simulink model "DTP_PMSM_VSD_Four_Vector_Control"  (R2024b)
settings: Solver=ode3  StartTime=0.0  StopTime=0.2  FixedStep=1e-6  RelTol=1e-3
InitFcn:
  | Udc=100;
  | Kp_omega = 2;
  | Ki_omega = 0;
  | 
  | Kp_id = 0.008*550;
  | Ki_id = 1.4*550;
  | Kp_iq = 0.008*550;
  | Ki_iq = 1.4*550;
  | Kp_z  = 0.1;
  | Ki_z  = 0.0001;
  | 
  | Ts = 1e-4;
  | flux = 0.015;
  | Toff = 1.02;
model workspace (MAT data in the model file):
  B = 0
  J = 0.000118
  Ki_id = 770
  Ki_iq = 770
  Ki_omega = 0
  Ki_z = 0.0001
  Kp_id = 4.4
  Kp_iq = 4.4
  Kp_omega = 2
  Kp_z = 0.1
  Lm = 1e-05
  Ls = 0.0001
  Pn = 5
  Rs = 0.28
  Toff = 1.02
  Ts = 0.0001
  Vdc = 100
  flux = 0.015
libraries: spsControlledVoltageSourceLib x6, spsCurrentMeasurementLib x6, powerlib_extras x5, spsUniversalBridgeLib x2, spsMutualInductanceLib x1, spsGroundLib x1, spsDCVoltageSourceLib x1, spspowerguiLib x1, simulink x1
settings Model: Creator=zx  LastModifiedBy=31904
settings SolverCC: AlgebraicLoopSolver=TrustRegion
settings DataIOCC: ReturnWorkspaceOutputs=off
settings DebuggingCC: ArithmeticOperatorsInVariantConditions=warning
settings SFSimCC: CustomCodeUndefinedFunction=UseInterfaceOnly
settings RTWCC: GPUComputeCapability=3.5

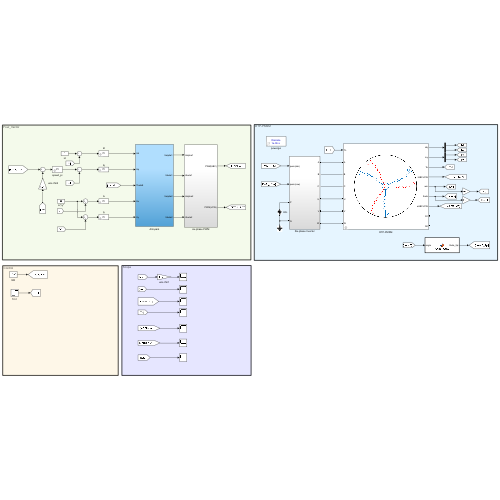
[thumbnail: Simulink's stored preview of the top-level diagram]
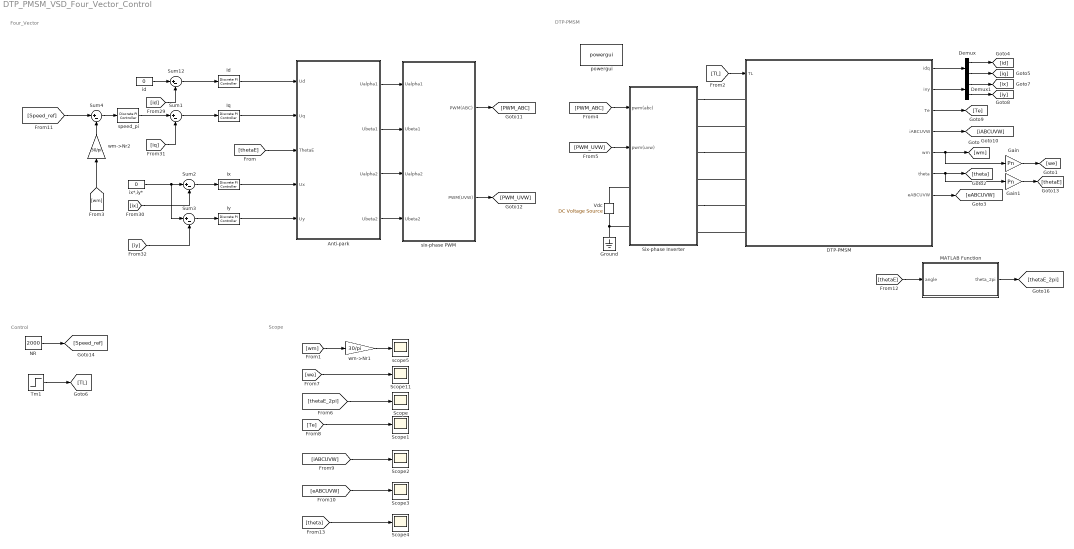
== system DTP_PMSM_VSD_Four_Vector_Control ==
  note: Four_Vector
  note: Control
  note: DTP-PMSM
  note: Scope
  Anti-park : Subsystem
  DTP-PMSM : Subsystem  mask{flux=flux, Ls=Ls, Lm=Lm, Rs=Rs, Inertia=J, Friction=B, Pairs=Pn}
      mask DialogControl ParameterGroupVar Prompt: DTP-PMSM Parameters
      mask Display: image('DTP-PMSM.png', [0,0,0,0,75,75]);
  Demux : Demux  Outputs=2
  Demux1 : Demux  Outputs=2
  Gain : Gain  Gain=Pn
  Gain1 : Gain  Gain=Pn
  Ground : spsGroundLib/Ground  LConnTagsString=a
  Id : powerlib_extras/Discrete  Control Blocks/Discrete PI Controller  Kp=0.111  Ki=280  Par_Limits=[Vdc*0.9*sqrt(1/3) -Vdc*0.9*sqrt(1/3)]  Init=0  Ts=Ts
  Iq : powerlib_extras/Discrete  Control Blocks/Discrete PI Controller  Kp=0.111  Ki=280  Par_Limits=[Vdc*0.9*sqrt(1/3) -Vdc*0.9*sqrt(1/3)]  Init=0  Ts=Ts
  Ix : powerlib_extras/Discrete  Control Blocks/Discrete PI Controller  Kp=Kp_z  Ki=Ki_z  Par_Limits=[100 -100]  Init=0  Ts=Ts
  Iy : powerlib_extras/Discrete  Control Blocks/Discrete PI Controller  Kp=Kp_z  Ki=Ki_z  Par_Limits=[100 -100]  Init=0  Ts=Ts
  MATLAB Function : MATLAB Function  TreatAsAtomicUnit=on
  NR : Constant  Value=2000
  Scope{,1..4,11} (6 alike) : Scope
  Six-phase Inverter : Subsystem
  Sum{1..4,12} (5 alike) : Sum  Inputs=|+-
  Tm1 : Step  Time=0.1  SampleTime=0
  Vdc : spsDCVoltageSourceLib/DC Voltage Source  Amplitude=Vdc  Measurements=None
  id : Constant  Value=0
  ix*,iy* : Constant  Value=0
  powergui : spspowerguiLib/powergui  Priority=1  SimulationMode=Discrete  SampleTime=1e-6  frequency=60  Iterations=50  frequencyindice=0  Pbase=100e6  ErrMax=1e-4  UnitsV=kV  UnitsW=MW  buscounter=0  FunctionMessages=off  echomessages=off  EnableUseOfTLC=off  CurrentSourceSwitches=off  DisableSnubberDevices=off  DisableRonSwitches=off  DisableVfSwitches=off  DisplayEquations=off  AutomaticDiscreteSolvers=off  SolverType=Tustin/Backward Euler (TBE)  Interpol=off  ExternalGateDelay=off  methode=off  Ts=100  x0status=blocks  SPID=on  SwTol=0  HookPort=off  NonlinearTolerance=1e-4  nMaxIteration=100  ContinueOnMaxIteration=off  RestoreLinks=warning  ResistiveCurrentMeasurement=off  Frange=[0:2:500]  Ylog=off  Xlog=on  ShowGrid=off  save=off  variable=ZData  structure=0  ZoomFFT=off  StartTime=0.0  cycles=1  DisplayStyle=1  fundamental=60  FreqAxis=off  MaxFrequency=1000  frequencyindicesteady=1  RmsSteady=1  display=off
  scope5 : Scope
  six-phase PWM : Subsystem
  speed_pi : powerlib_extras/Discrete  Control Blocks/Discrete PI Controller  Kp=0.03  Ki=1  Par_Limits=[50 -50]  Init=0  Ts=0.0001
  wm->Nr1 : Gain  Gain=30/pi
  wm->Nr2 : Gain  Gain=30/pi
  wires:
  [thetaE] -> Anti-park/3(ThetaE)
  Iq/1 -> Anti-park/2(Uq)
  [iq] -> Sum1/2
  id/1 -> Sum12/1
  Sum1/1 -> Iq/1
  Sum4/1 -> speed_pi/1
  Sum12/1 -> Id/1
  Ix/1 -> Anti-park/4(Ux)
  speed_pi/1 -> Sum1/1
  Id/1 -> Anti-park/1(Ud)
  Sum3/1 -> Iy/1
  NR/1 -> [Speed_ref]
  ix*,iy*/1 -> Sum3/1, Sum2/1
  Sum2/1 -> Ix/1
  Iy/1 -> Anti-park/5(Uy)
  [wm] -> wm->Nr2/1
  [wm] -> wm->Nr1/1
  wm->Nr1/1 -> scope5/1
  [ix] -> Sum2/2
  [iy] -> Sum3/2
  [id] -> Sum12/2
  Tm1/1 -> [TL]
  Anti-park/1(Ualpha1) -> six-phase PWM/1(Ualpha1)
  Anti-park/2(Ubeta1) -> six-phase PWM/2(Ubeta1)
  Anti-park/3(Ualpha2) -> six-phase PWM/3(Ualpha2)
  Anti-park/4(Ubeta2) -> six-phase PWM/4(Ubeta2)
  six-phase PWM/1(PWM(ABC)) -> [PWM_ABC]
  six-phase PWM/2(PWM(UVW)) -> [PWM_UVW]
  wm->Nr2/1 -> Sum4/2
  DTP-PMSM/4(iABCUVW) -> [iABCUVW]
  DTP-PMSM/3(Te) -> [Te]
  DTP-PMSM/2(ixy) -> Demux1/1
  DTP-PMSM/1(idq) -> Demux/1
  [we] -> Scope11/1
  DTP-PMSM/5(wm) -> Gain/1, [wm]
  Gain/1 -> [we]
  DTP-PMSM/6(theta) -> [theta], Gain1/1
  DTP-PMSM/7(eABCUVW) -> [eABCUVW]
  Demux/1 -> [id]
  Demux/2 -> [iq]
  [TL] -> DTP-PMSM/1(TL)
  Demux1/1 -> [ix]
  Demux1/2 -> [iy]
  [PWM_UVW] -> Six-phase Inverter/2(pwm(uvw))
  [PWM_ABC] -> Six-phase Inverter/1(pwm(abc))
  [Te] -> Scope1/1
  [iABCUVW] -> Scope2/1
  [eABCUVW] -> Scope3/1
  Gain1/1 -> [thetaE]
  [Speed_ref] -> Sum4/1
  [thetaE] -> MATLAB Function/1(angle)
  MATLAB Function/1(theta_2pi) -> [thetaE_2pi]
  [thetaE_2pi] -> Scope/1
  [theta] -> Scope4/1
  connections:
  DTP-PMSM/LConn4 -- Six-phase Inverter/RConn4
  Six-phase Inverter/RConn5 -- DTP-PMSM/LConn5
  Six-phase Inverter/RConn3 -- DTP-PMSM/LConn3
  DTP-PMSM/LConn2 -- Six-phase Inverter/RConn2
  Six-phase Inverter/RConn1 -- DTP-PMSM/LConn1
  DTP-PMSM/LConn6 -- Six-phase Inverter/RConn6
  Vdc/RConn1 -- Six-phase Inverter/LConn1
  Six-phase Inverter/LConn2 -- Vdc/LConn1 -- Ground/LConn1

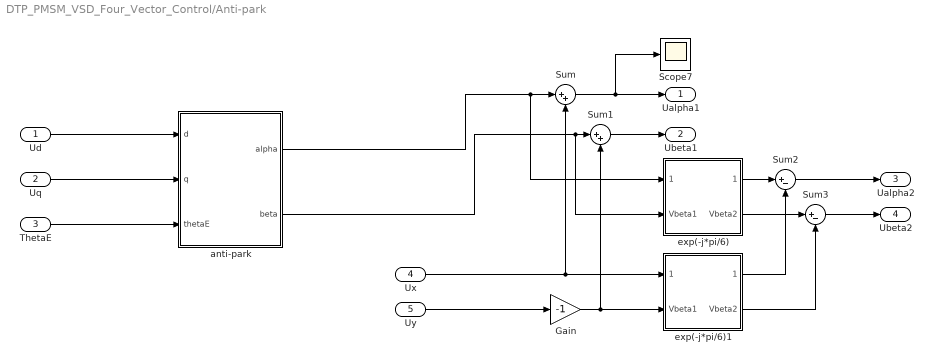
== system DTP_PMSM_VSD_Four_Vector_Control/Anti-park ==
  Ud : Inport
  Uq : Inport  Port=2
  ThetaE : Inport  Port=3
  Ux : Inport  Port=4
  Uy : Inport  Port=5
  Gain : Gain  Gain=-1
  Scope7 : Scope
  Sum : Sum  Inputs=|++
  Sum1 : Sum  Inputs=|++
  Sum2 : Sum  Inputs=|+-
  Sum3 : Sum  Inputs=|+-
  anti-park : Subsystem
      mask Display: disp('anti-park')
  exp(-j*pi/6) : Subsystem
  exp(-j*pi/6)1 : Subsystem
  Ualpha1 : Outport  VectorParamsAs1DForOutWhenUnconnected=off
  Ubeta1 : Outport  Port=2  VectorParamsAs1DForOutWhenUnconnected=off
  Ualpha2 : Outport  Port=3  VectorParamsAs1DForOutWhenUnconnected=off
  Ubeta2 : Outport  Port=4  VectorParamsAs1DForOutWhenUnconnected=off
  wires:
  ThetaE/1 -> anti-park/3(thetaE)
  Ud/1 -> anti-park/1(d)
  Uq/1 -> anti-park/2(q)
  Sum1/1 -> Ubeta1/1
  Sum3/1 -> Ubeta2/1
  Sum/1 -> Scope7/1, Ualpha1/1
  Sum2/1 -> Ualpha2/1
  Ux/1 -> Sum/2, exp(-j*pi/6)1/1(Valpha1)
  anti-park/2(beta) -> exp(-j*pi/6)/2(Vbeta1), Sum1/1
  exp(-j*pi/6)/2(Vbeta2) -> Sum3/1
  Gain/1 -> Sum1/2, exp(-j*pi/6)1/2(Vbeta1)
  Uy/1 -> Gain/1
  exp(-j*pi/6)/1(Valpha2) -> Sum2/1
  exp(-j*pi/6)1/1(Valpha2) -> Sum2/2
  exp(-j*pi/6)1/2(Vbeta2) -> Sum3/2
  anti-park/1(alpha) -> exp(-j*pi/6)/1(Valpha1), Sum/1

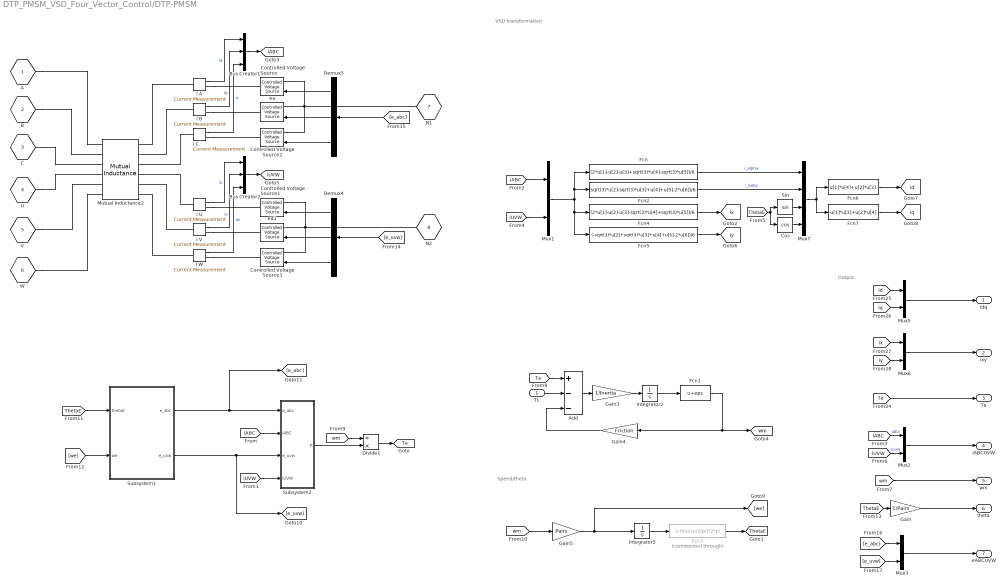
== system DTP_PMSM_VSD_Four_Vector_Control/DTP-PMSM ==
  note: Speed/theta
  note: Output
  note: VSD transformation
  TL : Inport
  Add : Sum  Inputs=+--
  Bus Creator1 : BusCreator  Inputs=3
  Bus Creator2 : BusCreator  Inputs=3
  Controlled Voltage Source{,1..3} (4 alike) : spsControlledVoltageSourceLib/Controlled Voltage Source  Initialize=on  Source_Type=AC  Amplitude=0  Phase=0  Frequency=0  Measurements=None
  Cos : Trigonometry  Operator=cos
  Demux3 : Demux  Outputs=3
  Demux4 : Demux  Outputs=3
  Divide1 : Product  Inputs=/*
  Fcn : Fcn  Expr=(2*u[1]-u[2]-u[3]+sqrt(3)*u[4]-sqrt(3)*u[5])/6
  Fcn1 : Fcn  Expr=u+eps
  Fcn2 : Fcn  Expr=(sqrt(3)*u[2]-sqrt(3)*u[3]+u[4]+u[5]-2*u[6])/6
  Fcn3 : Fcn  Commented=through  Expr=u-floor(u/2/pi)*2*pi
  Fcn4 : Fcn  Expr=(2*u[1]-u[2]-u[3]-sqrt(3)*u[4]+sqrt(3)*u[5])/6
  Fcn5 : Fcn  Expr=(-sqrt(3)*u[2]+sqrt(3)*u[3]+u[4]+u[5]-2*u[6])/6
  Fcn6 : Fcn  Expr=u[1]*u[4]+u[2]*u[3]
  Fcn7 : Fcn  Expr=-u[1]*u[3]+u[2]*u[4]
  Gain : Gain  Gain=1/Pairs
  Gain3 : Gain  Gain=1/Inertia
  Gain4 : Gain  Gain=Friction
  Gain5 : Gain  Gain=Pairs
  I A : spsCurrentMeasurementLib/Current Measurement  PhasorSimulation=off  OutputType=Complex  PSBequivalent=0
  I B : spsCurrentMeasurementLib/Current Measurement  PhasorSimulation=off  OutputType=Complex  PSBequivalent=0
  I C : spsCurrentMeasurementLib/Current Measurement  PhasorSimulation=off  OutputType=Complex  PSBequivalent=0
  I U : spsCurrentMeasurementLib/Current Measurement  PhasorSimulation=off  OutputType=Complex  PSBequivalent=0
  I V : spsCurrentMeasurementLib/Current Measurement  PhasorSimulation=off  OutputType=Complex  PSBequivalent=0
  I W : spsCurrentMeasurementLib/Current Measurement  PhasorSimulation=off  OutputType=Complex  PSBequivalent=0
  Integrator2 : Integrator  UpperSaturationLimit=100  LowerSaturationLimit=-100
  Integrator3 : Integrator
  Mutual Inductance2 : spsMutualInductanceLib/Mutual Inductance  LConnTagsString=a|b|c|L4|L5|L6  RConnTagsString=A|B|C|R4|R5|R6  TypeOfMutual=Generalized mutual inductance  NumberOfWindings=6  SelfImpedance1=[0.306 0.0016]  SelfImpedance2=[0.306 0.0016]  ThreeWindings=on  SelfImpedance3=[0.306 0.0016]  MutualImpedance=[0 0.0008]  InductanceMatrix=[Ls -Lm -Lm 1.732508*Lm -1.732508*Lm 0; -Lm Ls -Lm 0 1.732508*Lm -1.732508*Lm; -Lm -Lm Ls -1.732508*Lm 0 1.732508*Lm; 1.732508*Lm 0 -1.732508*Lm Ls -Lm -Lm; -1.732508*Lm 1.732508*Lm 0 -Lm Ls -Lm; 0 -1.732508*Lm 1.732508*Lm -Lm -Lm Ls]  ResistanceMatrix=[Rs 0 0 0 0 0; 0 Rs 0 0 0 0; 0 0 Rs 0 0 0; 0 0 0 Rs 0 0; 0 0 0 0 Rs 0; 0 0 0 0 0 Rs]  Measurements=None
      settings: LibrarySourceBlock=sps_lib/Passives/Mutual Inductance
  Mux{1..3,5..6} (5 alike) : Mux  Inputs=2
  Mux7 : Mux
  Sin : Trigonometry
  Subsystem1 : Subsystem
  Subsystem2 : Subsystem
  ea : spsControlledVoltageSourceLib/Controlled Voltage Source  Initialize=on  Source_Type=AC  Amplitude=0  Phase=0  Frequency=0  Measurements=None
  ea1 : spsControlledVoltageSourceLib/Controlled Voltage Source  Initialize=on  Source_Type=AC  Amplitude=0  Phase=0  Frequency=0  Measurements=None
  A : PMIOPort  Side=Left
  B : PMIOPort  Port=2  Side=Left
  C : PMIOPort  Port=3  Side=Left
  U : PMIOPort  Port=4  Side=Left
  V : PMIOPort  Port=5  Side=Left
  W : PMIOPort  Port=6  Side=Left
  N1 : PMIOPort  Port=7  Side=Right
  N2 : PMIOPort  Port=8  Side=Right
  idq : Outport  VectorParamsAs1DForOutWhenUnconnected=off
  ixy : Outport  Port=2  VectorParamsAs1DForOutWhenUnconnected=off
  Te : Outport  Port=3  VectorParamsAs1DForOutWhenUnconnected=off
  iABCUVW : Outport  Port=4  VectorParamsAs1DForOutWhenUnconnected=off
  wm : Outport  Port=5  VectorParamsAs1DForOutWhenUnconnected=off
  theta : Outport  Port=6  VectorParamsAs1DForOutWhenUnconnected=off
  eABCUVW : Outport  Port=7  VectorParamsAs1DForOutWhenUnconnected=off
  tag scope: Te=global, ThetaE=global, iABC=global, iUVW=global, id=global, iq=global, ix=global, iy=global, wm=global
  wires:
  Subsystem1/1(e_abc) -> [e_abc], Subsystem2/1(e_abc)
  Subsystem1/2(e_uvw) -> [e_uvw], Subsystem2/3(e_uvw)
  Demux3/1 -> Controlled Voltage Source/1
  Demux3/2 -> ea/1
  Demux3/3 -> Controlled Voltage Source2/1
  Demux4/1 -> Controlled Voltage Source1/1
  Demux4/2 -> ea1/1
  Demux4/3 -> Controlled Voltage Source3/1
  I A/1 -> Bus Creator1/1  "ia"
  I B/1 -> Bus Creator1/2  "ib"
  I C/1 -> Bus Creator1/3  "ic"
  I U/1 -> Bus Creator2/1  "iu"
  I V/1 -> Bus Creator2/2  "iv"
  I W/1 -> Bus Creator2/3  "iw"
  Bus Creator1/1 -> [iABC]
  Bus Creator2/1 -> [iUVW]
  [iABC] -> Subsystem2/2(iABC)
  [iUVW] -> Subsystem2/4(iUVW)
  Subsystem2/1(P) -> Divide1/2
  Divide1/1 -> [Te]
  TL/1 -> Add/2
  Add/1 -> Gain3/1
  Gain3/1 -> Integrator2/1
  Integrator2/1 -> Fcn1/1
  Fcn1/1 -> [wm], Gain4/1
  Gain4/1 -> Add/3
  Gain5/1 -> [we], Integrator3/1
  Integrator3/1 -> Fcn3/1
  Fcn3/1 -> [ThetaE]
  Fcn4/1 -> [ix]
  Mux1/1 -> Fcn2/1, Fcn/1, Fcn4/1, Fcn5/1
  [iUVW] -> Mux1/2
  Fcn7/1 -> [iq]
  [iABC] -> Mux1/1
  [ThetaE] -> Sin/1, Cos/1
  Fcn5/1 -> [iy]
  Fcn6/1 -> [id]
  Mux7/1 -> Fcn6/1, Fcn7/1
  Fcn2/1 -> Mux7/2  "i_beta"
  Fcn/1 -> Mux7/1  "i_alpha"
  Cos/1 -> Mux7/4
  Sin/1 -> Mux7/3
  Mux5/1 -> idq/1
  [id] -> Mux5/1
  Mux6/1 -> ixy/1
  [iy] -> Mux6/2
  [ix] -> Mux6/1
  [iq] -> Mux5/2
  [Te] -> Te/1
  [iABC] -> Mux2/1  "iabc"
  [iUVW] -> Mux2/2  "iuvw"
  [wm] -> wm/1
  Mux2/1 -> iABCUVW/1
  [Te] -> Add/1
  [wm] -> Divide1/1
  [wm] -> Gain5/1
  [ThetaE] -> Subsystem1/1(thetaE)
  [we] -> Subsystem1/2(we)
  [ThetaE] -> Gain/1
  Gain/1 -> theta/1
  [e_uvw] -> Demux4/1
  [e_abc] -> Demux3/1
  [e_abc] -> Mux3/1
  [e_uvw] -> Mux3/2
  Mux3/1 -> eABCUVW/1
  connections:
  N1/RConn1 -- Controlled Voltage Source/LConn1 -- ea/LConn1 -- Controlled Voltage Source2/LConn1
  I C/LConn1 -- Mutual Inductance2/RConn3
  A/RConn1 -- Mutual Inductance2/LConn1
  B/RConn1 -- Mutual Inductance2/LConn2
  C/RConn1 -- Mutual Inductance2/LConn3
  I B/RConn1 -- ea/RConn1
  I A/RConn1 -- Controlled Voltage Source/RConn1
  I B/LConn1 -- Mutual Inductance2/RConn2
  I C/RConn1 -- Controlled Voltage Source2/RConn1
  I A/LConn1 -- Mutual Inductance2/RConn1
  I U/RConn1 -- Controlled Voltage Source1/RConn1
  U/RConn1 -- Mutual Inductance2/LConn4
  I W/RConn1 -- Controlled Voltage Source3/RConn1
  I U/LConn1 -- Mutual Inductance2/RConn4
  I V/LConn1 -- Mutual Inductance2/RConn5
  Controlled Voltage Source3/LConn1 -- Controlled Voltage Source1/LConn1 -- ea1/LConn1 -- N2/RConn1
  V/RConn1 -- Mutual Inductance2/LConn5
  I V/RConn1 -- ea1/RConn1
  I W/LConn1 -- Mutual Inductance2/RConn6
  W/RConn1 -- Mutual Inductance2/LConn6

== system DTP_PMSM_VSD_Four_Vector_Control/Six-phase Inverter ==
  pwm(abc) : Inport
  pwm(uvw) : Inport  Port=2
  Universal Bridge : spsUniversalBridgeLib/Universal Bridge  Arms=3  SnubberResistance=1e5  SnubberCapacitance=inf  Device=IGBT / Diodes  Ron=1e-3  Lon=0  ForwardVoltages="[  0  0  ]"  ForwardVoltage=0  GTOparameters=[ 10e-6 , 20e-6 ]  IGBTparameters=[ 1e-6 , 2e-6 ]  Measurements=None  Measurements_2=None  converterType=Rectifier
  Universal Bridge1 : spsUniversalBridgeLib/Universal Bridge  Arms=3  SnubberResistance=1e5  SnubberCapacitance=inf  Device=IGBT / Diodes  Ron=1e-3  Lon=0  ForwardVoltages="[  0  0  ]"  ForwardVoltage=0  GTOparameters=[ 10e-6 , 20e-6 ]  IGBTparameters=[ 1e-6 , 2e-6 ]  Measurements=None  Measurements_2=None  converterType=Rectifier
  A : PMIOPort  Side=Right
  B : PMIOPort  Port=2  Side=Right
  C : PMIOPort  Port=3  Side=Right
  U : PMIOPort  Port=4  Side=Right
  V : PMIOPort  Port=5  Side=Right
  W : PMIOPort  Port=6  Side=Right
  P : PMIOPort  Port=7  Side=Left
  N : PMIOPort  Port=8  Side=Left
  wires:
  pwm(uvw)/1 -> Universal Bridge/1
  pwm(abc)/1 -> Universal Bridge1/1
  connections:
  Universal Bridge/RConn2 -- N/RConn1 -- Universal Bridge1/RConn2
  Universal Bridge/RConn1 -- P/RConn1 -- Universal Bridge1/RConn1
  V/RConn1 -- Universal Bridge/LConn2
  U/RConn1 -- Universal Bridge/LConn1
  B/RConn1 -- Universal Bridge1/LConn2
  W/RConn1 -- Universal Bridge/LConn3
  C/RConn1 -- Universal Bridge1/LConn3
  A/RConn1 -- Universal Bridge1/LConn1

== system DTP_PMSM_VSD_Four_Vector_Control/six-phase PWM ==
  Ualpha1 : Inport
  Ubeta1 : Inport  Port=2
  Ualpha2 : Inport  Port=3
  Ubeta2 : Inport  Port=4
  Repeating Sequence : simulink/Sources/Repeating Sequence  rep_seq_t=[0 Ts/2 Ts]  rep_seq_y=[0 Ts/2 0]
  SVPWM : Subsystem
  SVPWM1 : Subsystem
  PWM(ABC) : Outport
  PWM(UVW) : Outport  Port=2
  wires:
  SVPWM/1(Pulse) -> PWM(ABC)/1
  Ubeta1/1 -> SVPWM/2(Ubeta)
  Ualpha2/1 -> SVPWM1/1(Ualpha)
  SVPWM1/1(Pulse) -> PWM(UVW)/1
  Repeating Sequence/1 -> SVPWM/3(Carrier wave), SVPWM1/3(Carrier wave)
  Ualpha1/1 -> SVPWM/1(Ualpha)
  Ubeta2/1 -> SVPWM1/2(Ubeta)

== system DTP_PMSM_VSD_Four_Vector_Control/Anti-park/anti-park ==
  d : Inport
  q : Inport  Port=2
  thetaE : Inport  Port=3
  Fcn : Fcn  Expr=u[1]*u[4]-u[2]*u[3]
  Fcn1 : Fcn  Expr=u[1]*u[3]+u[2]*u[4]
  Mux2 : Mux
  cos : Trigonometry  Operator=cos
  sin : Trigonometry
  alpha : Outport  VectorParamsAs1DForOutWhenUnconnected=off
  beta : Outport  Port=2  VectorParamsAs1DForOutWhenUnconnected=off
  wires:
  d/1 -> Mux2/1
  sin/1 -> Mux2/3
  Mux2/1 -> Fcn1/1, Fcn/1
  q/1 -> Mux2/2
  thetaE/1 -> sin/1, cos/1
  Fcn1/1 -> beta/1
  cos/1 -> Mux2/4
  Fcn/1 -> alpha/1

== system DTP_PMSM_VSD_Four_Vector_Control/Anti-park/exp(-j*pi//6) ==
  Valpha1 : Inport
  Vbeta1 : Inport  Port=2
  Fcn : Fcn  Expr=u(1)*cos(pi/6)+u(2)*sin(pi/6)
  Fcn1 : Fcn  Expr=-u(1)*sin(pi/6)+u(2)*cos(pi/6)
  Mux : Mux  Inputs=2
  Valpha2 : Outport  VectorParamsAs1DForOutWhenUnconnected=off
  Vbeta2 : Outport  Port=2  VectorParamsAs1DForOutWhenUnconnected=off
  wires:
  Vbeta1/1 -> Mux/2
  Valpha1/1 -> Mux/1
  Mux/1 -> Fcn1/1, Fcn/1
  Fcn/1 -> Valpha2/1
  Fcn1/1 -> Vbeta2/1

== system DTP_PMSM_VSD_Four_Vector_Control/Anti-park/exp(-j*pi//6)1 ==
  Valpha1 : Inport
  Vbeta1 : Inport  Port=2
  Fcn : Fcn  Expr=u(1)*cos(pi/6)+u(2)*sin(pi/6)
  Fcn1 : Fcn  Expr=-u(1)*sin(pi/6)+u(2)*cos(pi/6)
  Mux : Mux  Inputs=2
  Valpha2 : Outport  VectorParamsAs1DForOutWhenUnconnected=off
  Vbeta2 : Outport  Port=2  VectorParamsAs1DForOutWhenUnconnected=off
  wires:
  Vbeta1/1 -> Mux/2
  Valpha1/1 -> Mux/1
  Mux/1 -> Fcn1/1, Fcn/1
  Fcn/1 -> Valpha2/1
  Fcn1/1 -> Vbeta2/1

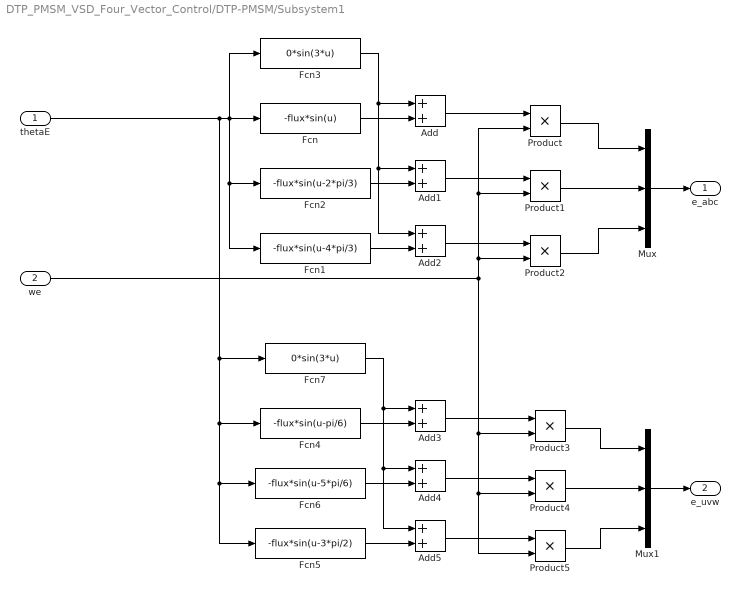
== system DTP_PMSM_VSD_Four_Vector_Control/DTP-PMSM/Subsystem1 ==
  thetaE : Inport
  we : Inport  Port=2
  Add{,1..5} (6 alike) : Sum
  Fcn : Fcn  Expr=-flux*sin(u)
  Fcn1 : Fcn  Expr=-flux*sin(u-4*pi/3)
  Fcn2 : Fcn  Expr=-flux*sin(u-2*pi/3)
  Fcn3 : Fcn  Expr=0*sin(3*u)
  Fcn4 : Fcn  Expr=-flux*sin(u-pi/6)
  Fcn5 : Fcn  Expr=-flux*sin(u-3*pi/2)
  Fcn6 : Fcn  Expr=-flux*sin(u-5*pi/6)
  Fcn7 : Fcn  Expr=0*sin(3*u)
  Mux : Mux  Inputs=3
  Mux1 : Mux  Inputs=3
  Product{,1..5} (6 alike) : Product
  e_abc : Outport
  e_uvw : Outport  Port=2
  wires:
  Product1/1 -> Mux/2
  Product2/1 -> Mux/3
  Mux/1 -> e_abc/1
  Product/1 -> Mux/1
  Fcn/1 -> Add/2
  Add/1 -> Product/1
  Fcn2/1 -> Add1/2
  Add1/1 -> Product1/1
  Fcn1/1 -> Add2/2
  Add2/1 -> Product2/1
  Fcn3/1 -> Add2/1, Add1/1, Add/1
  Product3/1 -> Mux1/1
  we/1 -> Product3/2, Product4/2, Product5/2, Product1/2, Product/2, Product2/2
  Product5/1 -> Mux1/3
  Add5/1 -> Product5/1
  Add4/1 -> Product4/1
  thetaE/1 -> Fcn5/1, Fcn6/1, Fcn4/1, Fcn7/1, Fcn1/1, Fcn2/1, Fcn3/1, Fcn/1
  Add3/1 -> Product3/1
  Fcn6/1 -> Add4/2
  Fcn4/1 -> Add3/2
  Product4/1 -> Mux1/2
  Fcn7/1 -> Add5/1, Add4/1, Add3/1
  Mux1/1 -> e_uvw/1
  Fcn5/1 -> Add5/2

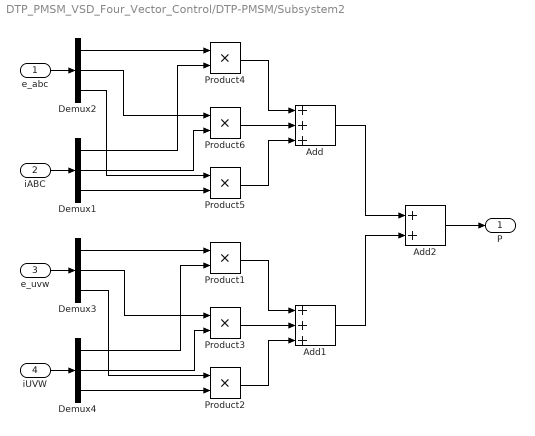
== system DTP_PMSM_VSD_Four_Vector_Control/DTP-PMSM/Subsystem2 ==
  e_abc : Inport
  iABC : Inport  Port=2
  e_uvw : Inport  Port=3
  iUVW : Inport  Port=4
  Add : Sum  Inputs=+++
  Add1 : Sum  Inputs=+++
  Add2 : Sum
  Demux{1..4} (4 alike) : Demux  Outputs=3
  Product{1..6} (6 alike) : Product
  P : Outport
  wires:
  e_abc/1 -> Demux2/1
  iABC/1 -> Demux1/1
  e_uvw/1 -> Demux3/1
  iUVW/1 -> Demux4/1
  Demux2/1 -> Product4/1
  Demux1/1 -> Product4/2
  Demux2/2 -> Product6/1
  Demux1/2 -> Product6/2
  Demux2/3 -> Product5/1
  Demux1/3 -> Product5/2
  Demux3/1 -> Product1/1
  Demux3/2 -> Product3/1
  Demux3/3 -> Product2/1
  Demux4/1 -> Product1/2
  Demux4/2 -> Product3/2
  Demux4/3 -> Product2/2
  Product6/1 -> Add/2
  Product4/1 -> Add/1
  Product5/1 -> Add/3
  Product3/1 -> Add1/2
  Product1/1 -> Add1/1
  Product2/1 -> Add1/3
  Add/1 -> Add2/1
  Add1/1 -> Add2/2
  Add2/1 -> P/1

== system DTP_PMSM_VSD_Four_Vector_Control/six-phase PWM/SVPWM ==
  Ualpha : Inport
  Ubeta : Inport  Port=2
  Carrier wave : Inport  Port=3
  PWM : Subsystem
  Sector Caculate : Subsystem
  T1T2 Caculate : Subsystem
  Tcm Caculate : Subsystem
  Tpwm : Constant  Value=Ts
  Vdc : Constant  Value=Vdc
  XYZ Caculate : Subsystem
  Pulse : Outport  VectorParamsAs1DForOutWhenUnconnected=off
  wires:
  Tcm Caculate/1(Tcm123) -> PWM/2(Tcm123)
  Carrier wave/1 -> PWM/1(In)
  PWM/1(PWM) -> Pulse/1
  Vdc/1 -> XYZ Caculate/4(Udc)
  Tpwm/1 -> XYZ Caculate/3(Ts), T1T2 Caculate/3(Tpwm), Tcm Caculate/4(Tpwm)
  T1T2 Caculate/2(T2) -> Tcm Caculate/3(T2)
  T1T2 Caculate/1(T1) -> Tcm Caculate/2(T1)
  XYZ Caculate/1(XYZ) -> T1T2 Caculate/2(XYZ)
  Sector Caculate/1(N) -> T1T2 Caculate/1(N), Tcm Caculate/1(N)
  Ubeta/1 -> Sector Caculate/2(Ubeta), XYZ Caculate/2(Ubeta)
  Ualpha/1 -> Sector Caculate/1(Ualpha), XYZ Caculate/1(Ualpha)

== system DTP_PMSM_VSD_Four_Vector_Control/six-phase PWM/SVPWM1 ==
  Ualpha : Inport
  Ubeta : Inport  Port=2
  Carrier wave : Inport  Port=3
  PWM : Subsystem
  Sector Caculate : Subsystem
  T1T2 Caculate : Subsystem
  Tcm Caculate : Subsystem
  Tpwm : Constant  Value=Ts
  Vdc : Constant  Value=Vdc
  XYZ Caculate : Subsystem
  Pulse : Outport  VectorParamsAs1DForOutWhenUnconnected=off
  wires:
  Tcm Caculate/1(Tcm123) -> PWM/2(Tcm123)
  Carrier wave/1 -> PWM/1(In)
  Ualpha/1 -> XYZ Caculate/1(Ualpha), Sector Caculate/1(Ualpha)
  Ubeta/1 -> XYZ Caculate/2(Ubeta), Sector Caculate/2(Ubeta)
  Sector Caculate/1(N) -> Tcm Caculate/1(N), T1T2 Caculate/1(N)
  XYZ Caculate/1(XYZ) -> T1T2 Caculate/2(XYZ)
  T1T2 Caculate/1(T1) -> Tcm Caculate/2(T1)
  T1T2 Caculate/2(T2) -> Tcm Caculate/3(T2)
  Tpwm/1 -> Tcm Caculate/4(Tpwm), T1T2 Caculate/3(Tpwm), XYZ Caculate/3(Ts)
  Vdc/1 -> XYZ Caculate/4(Udc)
  PWM/1(PWM) -> Pulse/1

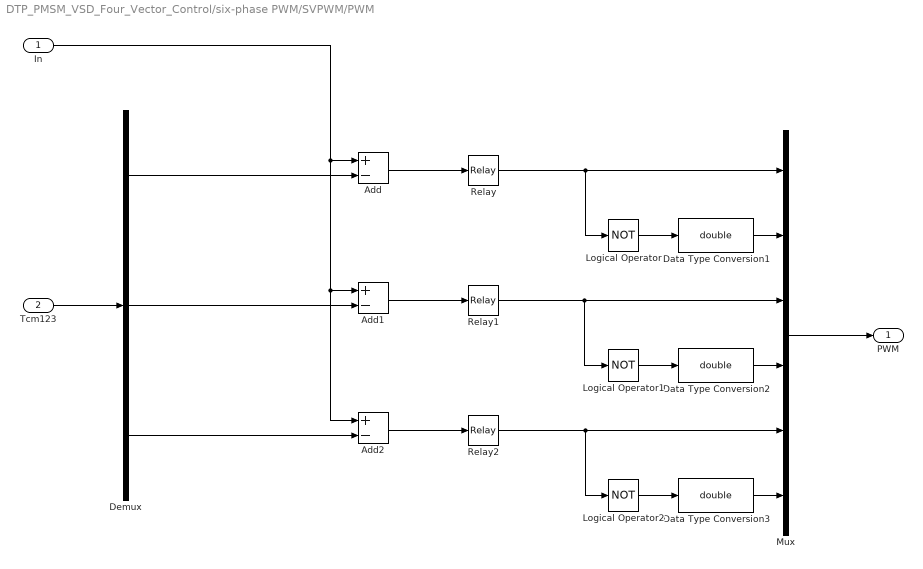
== system DTP_PMSM_VSD_Four_Vector_Control/six-phase PWM/SVPWM/PWM ==
  In : Inport
  Tcm123 : Inport  Port=2
  Add : Sum  Inputs=+-
  Add1 : Sum  Inputs=+-
  Add2 : Sum  Inputs=+-
  Data Type Conversion1 : DataTypeConversion  OutDataTypeStr=double
  Data Type Conversion2 : DataTypeConversion  OutDataTypeStr=double
  Data Type Conversion3 : DataTypeConversion  OutDataTypeStr=double
  Demux : Demux  Outputs=3
  Logical Operator : Logic  Operator=NOT  AllPortsSameDT=off  OutDataTypeStr=boolean
  Logical Operator1 : Logic  Operator=NOT  AllPortsSameDT=off  OutDataTypeStr=boolean
  Logical Operator2 : Logic  Operator=NOT  AllPortsSameDT=off  OutDataTypeStr=boolean
  Mux : Mux  Inputs=6
  Relay : Relay
  Relay1 : Relay
  Relay2 : Relay
  PWM : Outport  VectorParamsAs1DForOutWhenUnconnected=off
  wires:
  Data Type Conversion3/1 -> Mux/6
  Logical Operator2/1 -> Data Type Conversion3/1
  Data Type Conversion2/1 -> Mux/4
  Logical Operator1/1 -> Data Type Conversion2/1
  Data Type Conversion1/1 -> Mux/2
  Logical Operator/1 -> Data Type Conversion1/1
  Demux/3 -> Add2/2
  Demux/2 -> Add1/2
  Demux/1 -> Add/2
  Relay2/1 -> Logical Operator2/1, Mux/5
  Relay1/1 -> Mux/3, Logical Operator1/1
  Relay/1 -> Logical Operator/1, Mux/1
  Tcm123/1 -> Demux/1
  Add2/1 -> Relay2/1
  Add1/1 -> Relay1/1
  Add/1 -> Relay/1
  Mux/1 -> PWM/1
  In/1 -> Add1/1, Add2/1, Add/1

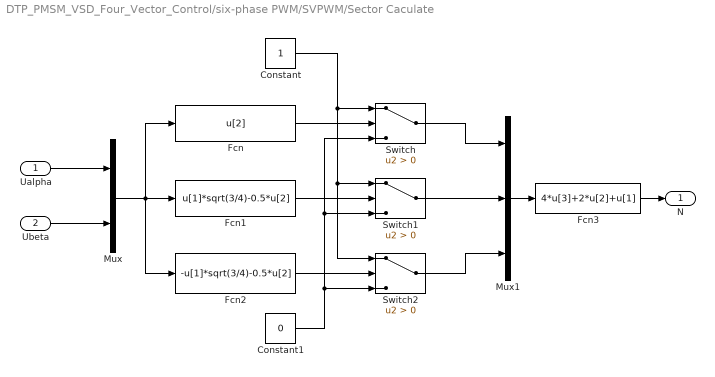
== system DTP_PMSM_VSD_Four_Vector_Control/six-phase PWM/SVPWM/Sector Caculate ==
  Ualpha : Inport
  Ubeta : Inport  Port=2
  Constant : Constant
  Constant1 : Constant  Value=0
  Fcn : Fcn  Expr=u[2]
  Fcn1 : Fcn  Expr=u[1]*sqrt(3/4)-0.5*u[2]
  Fcn2 : Fcn  Expr=-u[1]*sqrt(3/4)-0.5*u[2]
  Fcn3 : Fcn  Expr=4*u[3]+2*u[2]+u[1]
  Mux : Mux  Inputs=2
  Mux1 : Mux  Inputs=3
  Switch : Switch  Criteria=u2 > Threshold  SaturateOnIntegerOverflow=off  InputSameDT=off
  Switch1 : Switch  Criteria=u2 > Threshold  SaturateOnIntegerOverflow=off  InputSameDT=off
  Switch2 : Switch  Criteria=u2 > Threshold  SaturateOnIntegerOverflow=off  InputSameDT=off
  N : Outport  VectorParamsAs1DForOutWhenUnconnected=off
  wires:
  Constant1/1 -> Switch2/3, Switch1/3, Switch/3
  Constant/1 -> Switch/1, Switch2/1, Switch1/1
  Fcn2/1 -> Switch2/2
  Fcn1/1 -> Switch1/2
  Fcn/1 -> Switch/2
  Mux/1 -> Fcn/1, Fcn1/1, Fcn2/1
  Switch/1 -> Mux1/1
  Switch2/1 -> Mux1/3
  Switch1/1 -> Mux1/2
  Mux1/1 -> Fcn3/1
  Fcn3/1 -> N/1
  Ubeta/1 -> Mux/2
  Ualpha/1 -> Mux/1

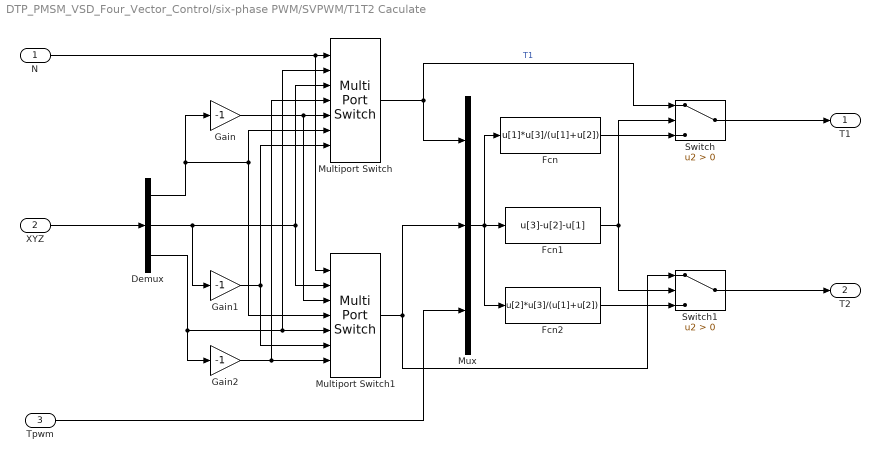
== system DTP_PMSM_VSD_Four_Vector_Control/six-phase PWM/SVPWM/T1T2 Caculate ==
  N : Inport
  XYZ : Inport  Port=2
  Tpwm : Inport  Port=3
  Demux : Demux  Outputs=3
  Fcn : Fcn  Expr=u[1]*u[3]/(u[1]+u[2])
  Fcn1 : Fcn  Expr=u[3]-u[2]-u[1]
  Fcn2 : Fcn  Expr=u[2]*u[3]/(u[1]+u[2])
  Gain : Gain  Gain=-1
  Gain1 : Gain  Gain=-1
  Gain2 : Gain  Gain=-1
  Multiport Switch : MultiPortSwitch  Inputs=6  DiagnosticForDefault=None  SaturateOnIntegerOverflow=off  InputSameDT=off
  Multiport Switch1 : MultiPortSwitch  Inputs=6  DiagnosticForDefault=None  SaturateOnIntegerOverflow=off  InputSameDT=off
  Mux : Mux  Inputs=3
  Switch : Switch  Criteria=u2 > Threshold  SaturateOnIntegerOverflow=off  InputSameDT=off
  Switch1 : Switch  Criteria=u2 > Threshold  SaturateOnIntegerOverflow=off  InputSameDT=off
  T1 : Outport  VectorParamsAs1DForOutWhenUnconnected=off
  T2 : Outport  Port=2  VectorParamsAs1DForOutWhenUnconnected=off
  wires:
  Switch1/1 -> T2/1
  Fcn2/1 -> Switch1/3
  Fcn1/1 -> Switch/2, Switch1/2
  Mux/1 -> Fcn/1, Fcn1/1, Fcn2/1
  Switch/1 -> T1/1
  Fcn/1 -> Switch/3
  Gain/1 -> Multiport Switch1/3, Multiport Switch/5
  Gain1/1 -> Multiport Switch/7, Multiport Switch1/6
  Gain2/1 -> Multiport Switch1/7, Multiport Switch/4
  Multiport Switch/1 -> Switch/1, Mux/1  "T1"
  Multiport Switch1/1 -> Mux/2, Switch1/1
  Tpwm/1 -> Mux/3
  Demux/3 -> Multiport Switch1/5, Multiport Switch/2, Gain2/1
  Demux/1 -> Multiport Switch/6, Multiport Switch1/4, Gain/1
  N/1 -> Multiport Switch/1, Multiport Switch1/1
  Demux/2 -> Gain1/1, Multiport Switch/3, Multiport Switch1/2
  XYZ/1 -> Demux/1

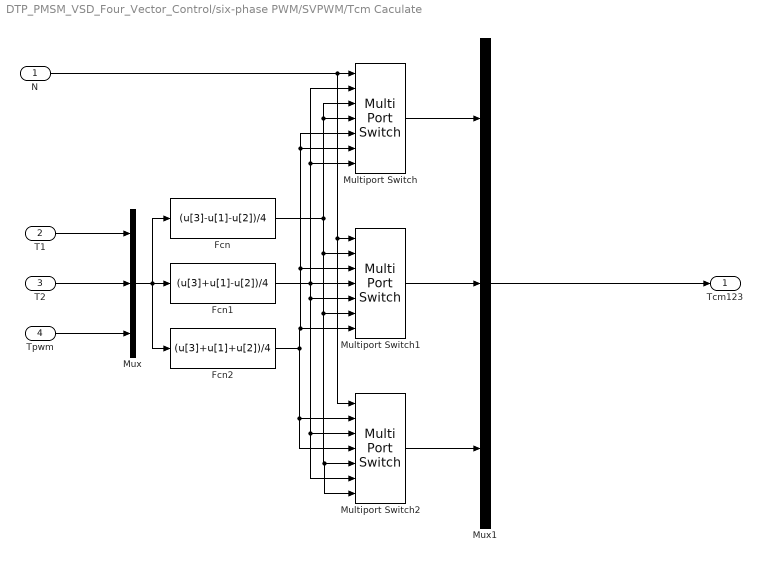
== system DTP_PMSM_VSD_Four_Vector_Control/six-phase PWM/SVPWM/Tcm Caculate ==
  N : Inport
  T1 : Inport  Port=2
  T2 : Inport  Port=3
  Tpwm : Inport  Port=4
  Fcn : Fcn  Expr=(u[3]-u[1]-u[2])/4
  Fcn1 : Fcn  Expr=(u[3]+u[1]-u[2])/4
  Fcn2 : Fcn  Expr=(u[3]+u[1]+u[2])/4
  Multiport Switch : MultiPortSwitch  Inputs=6  DiagnosticForDefault=None  SaturateOnIntegerOverflow=off  InputSameDT=off
  Multiport Switch1 : MultiPortSwitch  Inputs=6  DiagnosticForDefault=None  SaturateOnIntegerOverflow=off  InputSameDT=off
  Multiport Switch2 : MultiPortSwitch  Inputs=6  DiagnosticForDefault=None  SaturateOnIntegerOverflow=off  InputSameDT=off
  Mux : Mux  Inputs=3
  Mux1 : Mux  Inputs=3
  Tcm123 : Outport  VectorParamsAs1DForOutWhenUnconnected=off
  wires:
  Multiport Switch/1 -> Mux1/1
  Multiport Switch1/1 -> Mux1/2
  Multiport Switch2/1 -> Mux1/3
  Fcn2/1 -> Multiport Switch1/7, Multiport Switch1/3, Multiport Switch/6, Multiport Switch/5, Multiport Switch2/2, Multiport Switch2/4
  Fcn1/1 -> Multiport Switch1/4, Multiport Switch/7, Multiport Switch/2, Multiport Switch2/3, Multiport Switch2/6, Multiport Switch1/5
  Fcn/1 -> Multiport Switch1/2, Multiport Switch1/6, Multiport Switch2/5, Multiport Switch2/7, Multiport Switch/4, Multiport Switch/3
  Mux1/1 -> Tcm123/1
  Mux/1 -> Fcn1/1, Fcn2/1, Fcn/1
  Tpwm/1 -> Mux/3
  T2/1 -> Mux/2
  T1/1 -> Mux/1
  N/1 -> Multiport Switch/1, Multiport Switch1/1, Multiport Switch2/1

== system DTP_PMSM_VSD_Four_Vector_Control/six-phase PWM/SVPWM/XYZ Caculate ==
  Ualpha : Inport
  Ubeta : Inport  Port=2
  Ts : Inport  Port=3
  Udc : Inport  Port=4
  Fcn : Fcn  Expr=(sqrt(3)*u[3]*u[2])/u[4]
  Fcn1 : Fcn  Expr=sqrt(3)*u[3]*(sqrt(3)*u[1]+u[2])/(2*u[4])
  Fcn3 : Fcn  Expr=sqrt(3)*u[3]*(-sqrt(3)*u[1]+u[2])/(2*u[4])
  Mux : Mux  Inputs=3
  Mux1 : Mux
  XYZ : Outport  VectorParamsAs1DForOutWhenUnconnected=off
  wires:
  Fcn3/1 -> Mux/3
  Fcn1/1 -> Mux/2
  Fcn/1 -> Mux/1
  Mux1/1 -> Fcn/1, Fcn1/1, Fcn3/1
  Ts/1 -> Mux1/3
  Ubeta/1 -> Mux1/2
  Ualpha/1 -> Mux1/1
  Udc/1 -> Mux1/4
  Mux/1 -> XYZ/1

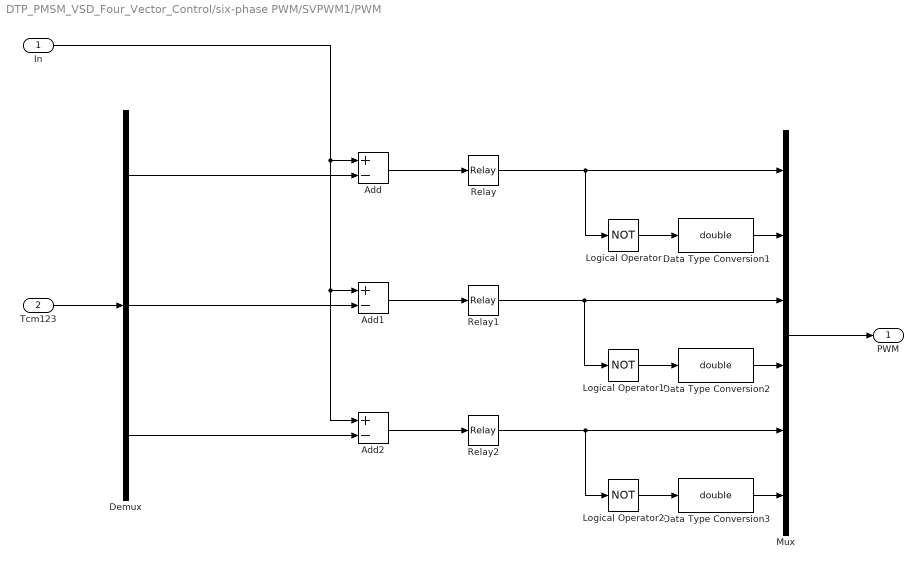
== system DTP_PMSM_VSD_Four_Vector_Control/six-phase PWM/SVPWM1/PWM ==
  In : Inport
  Tcm123 : Inport  Port=2
  Add : Sum  Inputs=+-
  Add1 : Sum  Inputs=+-
  Add2 : Sum  Inputs=+-
  Data Type Conversion1 : DataTypeConversion  OutDataTypeStr=double
  Data Type Conversion2 : DataTypeConversion  OutDataTypeStr=double
  Data Type Conversion3 : DataTypeConversion  OutDataTypeStr=double
  Demux : Demux  Outputs=3
  Logical Operator : Logic  Operator=NOT  AllPortsSameDT=off  OutDataTypeStr=boolean
  Logical Operator1 : Logic  Operator=NOT  AllPortsSameDT=off  OutDataTypeStr=boolean
  Logical Operator2 : Logic  Operator=NOT  AllPortsSameDT=off  OutDataTypeStr=boolean
  Mux : Mux  Inputs=6
  Relay : Relay
  Relay1 : Relay
  Relay2 : Relay
  PWM : Outport  VectorParamsAs1DForOutWhenUnconnected=off
  wires:
  In/1 -> Add/1, Add2/1, Add1/1
  Mux/1 -> PWM/1
  Add/1 -> Relay/1
  Add1/1 -> Relay1/1
  Add2/1 -> Relay2/1
  Tcm123/1 -> Demux/1
  Relay/1 -> Mux/1, Logical Operator/1
  Relay1/1 -> Logical Operator1/1, Mux/3
  Relay2/1 -> Mux/5, Logical Operator2/1
  Demux/1 -> Add/2
  Demux/2 -> Add1/2
  Demux/3 -> Add2/2
  Logical Operator/1 -> Data Type Conversion1/1
  Data Type Conversion1/1 -> Mux/2
  Logical Operator1/1 -> Data Type Conversion2/1
  Data Type Conversion2/1 -> Mux/4
  Logical Operator2/1 -> Data Type Conversion3/1
  Data Type Conversion3/1 -> Mux/6

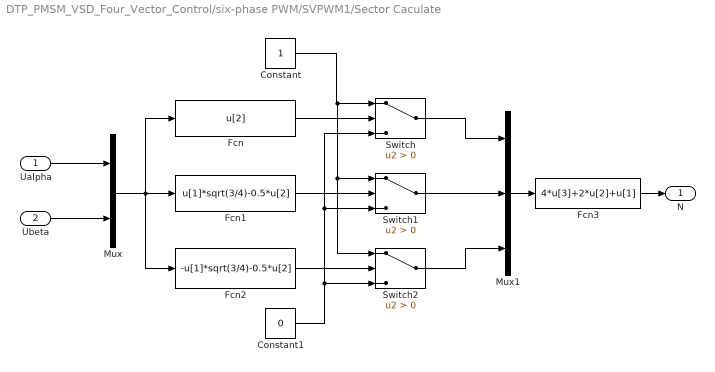
== system DTP_PMSM_VSD_Four_Vector_Control/six-phase PWM/SVPWM1/Sector Caculate ==
  Ualpha : Inport
  Ubeta : Inport  Port=2
  Constant : Constant
  Constant1 : Constant  Value=0
  Fcn : Fcn  Expr=u[2]
  Fcn1 : Fcn  Expr=u[1]*sqrt(3/4)-0.5*u[2]
  Fcn2 : Fcn  Expr=-u[1]*sqrt(3/4)-0.5*u[2]
  Fcn3 : Fcn  Expr=4*u[3]+2*u[2]+u[1]
  Mux : Mux  Inputs=2
  Mux1 : Mux  Inputs=3
  Switch : Switch  Criteria=u2 > Threshold  SaturateOnIntegerOverflow=off  InputSameDT=off
  Switch1 : Switch  Criteria=u2 > Threshold  SaturateOnIntegerOverflow=off  InputSameDT=off
  Switch2 : Switch  Criteria=u2 > Threshold  SaturateOnIntegerOverflow=off  InputSameDT=off
  N : Outport  VectorParamsAs1DForOutWhenUnconnected=off
  wires:
  Ualpha/1 -> Mux/1
  Ubeta/1 -> Mux/2
  Fcn3/1 -> N/1
  Mux1/1 -> Fcn3/1
  Switch1/1 -> Mux1/2
  Switch2/1 -> Mux1/3
  Switch/1 -> Mux1/1
  Mux/1 -> Fcn2/1, Fcn1/1, Fcn/1
  Fcn/1 -> Switch/2
  Fcn1/1 -> Switch1/2
  Fcn2/1 -> Switch2/2
  Constant/1 -> Switch1/1, Switch2/1, Switch/1
  Constant1/1 -> Switch/3, Switch1/3, Switch2/3

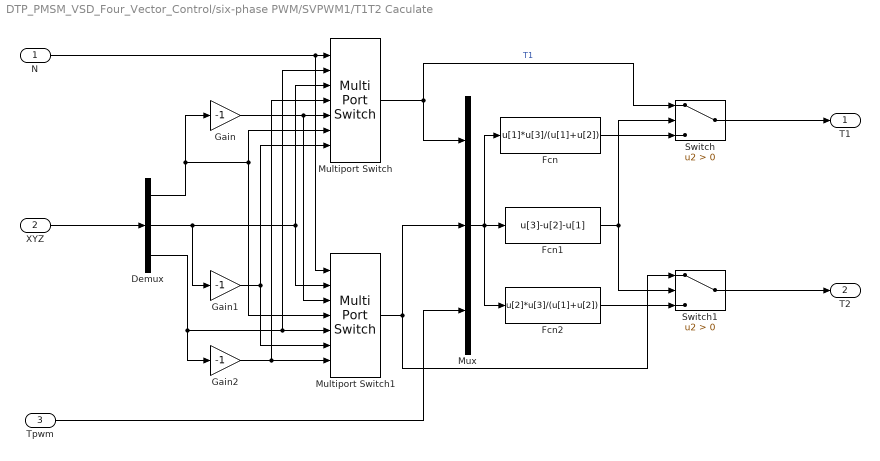
== system DTP_PMSM_VSD_Four_Vector_Control/six-phase PWM/SVPWM1/T1T2 Caculate ==
  N : Inport
  XYZ : Inport  Port=2
  Tpwm : Inport  Port=3
  Demux : Demux  Outputs=3
  Fcn : Fcn  Expr=u[1]*u[3]/(u[1]+u[2])
  Fcn1 : Fcn  Expr=u[3]-u[2]-u[1]
  Fcn2 : Fcn  Expr=u[2]*u[3]/(u[1]+u[2])
  Gain : Gain  Gain=-1
  Gain1 : Gain  Gain=-1
  Gain2 : Gain  Gain=-1
  Multiport Switch : MultiPortSwitch  Inputs=6  DiagnosticForDefault=None  SaturateOnIntegerOverflow=off  InputSameDT=off
  Multiport Switch1 : MultiPortSwitch  Inputs=6  DiagnosticForDefault=None  SaturateOnIntegerOverflow=off  InputSameDT=off
  Mux : Mux  Inputs=3
  Switch : Switch  Criteria=u2 > Threshold  SaturateOnIntegerOverflow=off  InputSameDT=off
  Switch1 : Switch  Criteria=u2 > Threshold  SaturateOnIntegerOverflow=off  InputSameDT=off
  T1 : Outport  VectorParamsAs1DForOutWhenUnconnected=off
  T2 : Outport  Port=2  VectorParamsAs1DForOutWhenUnconnected=off
  wires:
  XYZ/1 -> Demux/1
  Demux/2 -> Multiport Switch1/2, Multiport Switch/3, Gain1/1
  N/1 -> Multiport Switch1/1, Multiport Switch/1
  Demux/1 -> Gain/1, Multiport Switch1/4, Multiport Switch/6
  Demux/3 -> Gain2/1, Multiport Switch/2, Multiport Switch1/5
  Tpwm/1 -> Mux/3
  Multiport Switch1/1 -> Switch1/1, Mux/2
  Multiport Switch/1 -> Mux/1, Switch/1  "T1"
  Gain2/1 -> Multiport Switch/4, Multiport Switch1/7
  Gain1/1 -> Multiport Switch1/6, Multiport Switch/7
  Gain/1 -> Multiport Switch/5, Multiport Switch1/3
  Fcn/1 -> Switch/3
  Switch/1 -> T1/1
  Mux/1 -> Fcn2/1, Fcn1/1, Fcn/1
  Fcn1/1 -> Switch1/2, Switch/2
  Fcn2/1 -> Switch1/3
  Switch1/1 -> T2/1

== system DTP_PMSM_VSD_Four_Vector_Control/six-phase PWM/SVPWM1/Tcm Caculate ==
  N : Inport
  T1 : Inport  Port=2
  T2 : Inport  Port=3
  Tpwm : Inport  Port=4
  Fcn : Fcn  Expr=(u[3]-u[1]-u[2])/4
  Fcn1 : Fcn  Expr=(u[3]+u[1]-u[2])/4
  Fcn2 : Fcn  Expr=(u[3]+u[1]+u[2])/4
  Multiport Switch : MultiPortSwitch  Inputs=6  DiagnosticForDefault=None  SaturateOnIntegerOverflow=off  InputSameDT=off
  Multiport Switch1 : MultiPortSwitch  Inputs=6  DiagnosticForDefault=None  SaturateOnIntegerOverflow=off  InputSameDT=off
  Multiport Switch2 : MultiPortSwitch  Inputs=6  DiagnosticForDefault=None  SaturateOnIntegerOverflow=off  InputSameDT=off
  Mux : Mux  Inputs=3
  Mux1 : Mux  Inputs=3
  Tcm123 : Outport  VectorParamsAs1DForOutWhenUnconnected=off
  wires:
  N/1 -> Multiport Switch2/1, Multiport Switch1/1, Multiport Switch/1
  T1/1 -> Mux/1
  T2/1 -> Mux/2
  Tpwm/1 -> Mux/3
  Mux/1 -> Fcn/1, Fcn2/1, Fcn1/1
  Mux1/1 -> Tcm123/1
  Fcn/1 -> Multiport Switch/3, Multiport Switch/4, Multiport Switch2/7, Multiport Switch2/5, Multiport Switch1/6, Multiport Switch1/2
  Fcn1/1 -> Multiport Switch1/5, Multiport Switch2/6, Multiport Switch2/3, Multiport Switch/2, Multiport Switch/7, Multiport Switch1/4
  Fcn2/1 -> Multiport Switch2/4, Multiport Switch2/2, Multiport Switch/5, Multiport Switch/6, Multiport Switch1/3, Multiport Switch1/7
  Multiport Switch2/1 -> Mux1/3
  Multiport Switch1/1 -> Mux1/2
  Multiport Switch/1 -> Mux1/1

== system DTP_PMSM_VSD_Four_Vector_Control/six-phase PWM/SVPWM1/XYZ Caculate ==
  Ualpha : Inport
  Ubeta : Inport  Port=2
  Ts : Inport  Port=3
  Udc : Inport  Port=4
  Fcn : Fcn  Expr=(sqrt(3)*u[3]*u[2])/u[4]
  Fcn1 : Fcn  Expr=sqrt(3)*u[3]*(sqrt(3)*u[1]+u[2])/(2*u[4])
  Fcn3 : Fcn  Expr=sqrt(3)*u[3]*(-sqrt(3)*u[1]+u[2])/(2*u[4])
  Mux : Mux  Inputs=3
  Mux1 : Mux
  XYZ : Outport  VectorParamsAs1DForOutWhenUnconnected=off
  wires:
  Mux/1 -> XYZ/1
  Udc/1 -> Mux1/4
  Ualpha/1 -> Mux1/1
  Ubeta/1 -> Mux1/2
  Ts/1 -> Mux1/3
  Mux1/1 -> Fcn3/1, Fcn1/1, Fcn/1
  Fcn/1 -> Mux/1
  Fcn1/1 -> Mux/2
  Fcn3/1 -> Mux/3

== matlab function DTP_PMSM_VSD_Four_Vector_Control/MATLAB Function ==
  data: angle input; theta_2pi output
function theta_2pi = Angle_Conv(angle)

theta_2pi=mod(angle,2*pi);
